simulink model "nonlinear_dynamics_block"  (R2024b)
settings: Solver=VariableStepAuto  StartTime=0.0  StopTime=10.0  RelTol=1e-3
undefined symbols (not defined in the file): K
settings Model: Creator=kaleb  LastModifiedBy=kaleb
settings DataIOCC: ExternalInput=getinputstruct(op_trim1)  InitialState=getstatestruct(op_trim1)

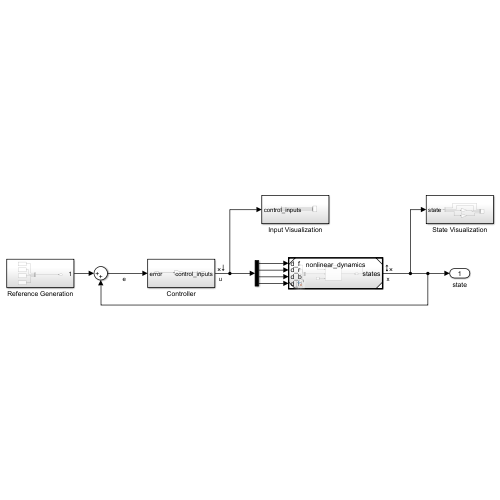
[thumbnail: Simulink's stored preview of the top-level diagram]
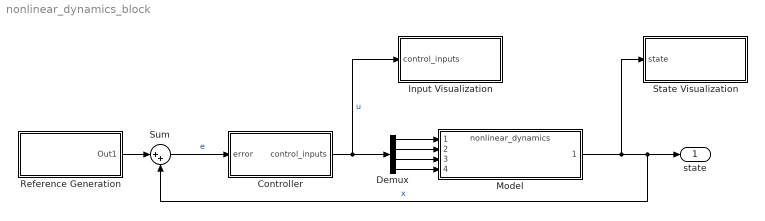
== system nonlinear_dynamics_block ==
  Controller : Subsystem
  Demux : Demux
  Input Visualization : Subsystem
  Model : ModelReference  ModelNameDialog=nonlinear_dynamics.slx  ModelReferenceVersion=1.2
  Reference Generation : Subsystem
  State Visualization : Subsystem
  Sum : Sum  Inputs=|++
  state : Outport
  wires:
  Sum/1 -> Controller/1(error)  "e"
  Reference Generation/1(Out1) -> Sum/1
  Model/1 -> State Visualization/1(state), state/1, Sum/2  "x"
  Controller/1(control_inputs) -> Input Visualization/1(control_inputs), Demux/1  "u"
  Demux/3 -> Model/3
  Demux/4 -> Model/4
  Demux/2 -> Model/2
  Demux/1 -> Model/1

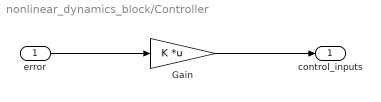
== system nonlinear_dynamics_block/Controller ==
  error : Inport
  Gain : Gain  Gain=K  Multiplication=Matrix(K*u)
  control_inputs : Outport
  wires:
  error/1 -> Gain/1
  Gain/1 -> control_inputs/1

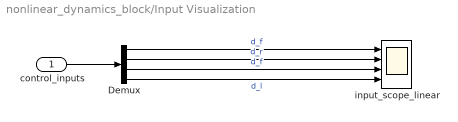
== system nonlinear_dynamics_block/Input Visualization ==
  control_inputs : Inport
  Demux : Demux
  input_scope_linear : Scope  NumInputPorts=4
  wires:
  Demux/4 -> input_scope_linear/4  "d_l"
  Demux/1 -> input_scope_linear/1  "d_f"
  Demux/2 -> input_scope_linear/2  "d_r"
  Demux/3 -> input_scope_linear/3  "d_f"
  control_inputs/1 -> Demux/1

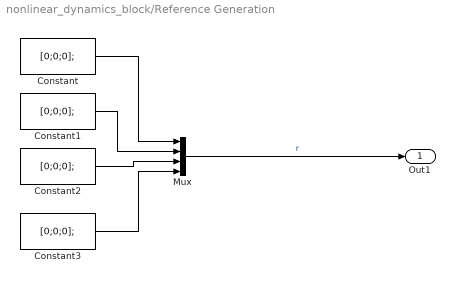
== system nonlinear_dynamics_block/Reference Generation ==
  Constant{,1..3} (4 alike) : Constant  Value=[0;0;0];
  Mux : Mux
  Out1 : Outport
  wires:
  Mux/1 -> Out1/1  "r"
  Constant/1 -> Mux/1
  Constant1/1 -> Mux/2
  Constant2/1 -> Mux/3
  Constant3/1 -> Mux/4

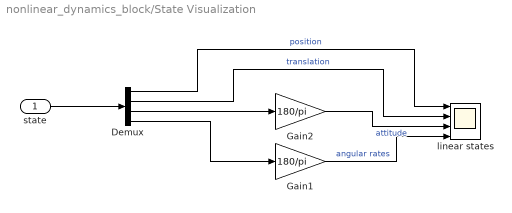
== system nonlinear_dynamics_block/State Visualization ==
  state : Inport
  Demux : Demux
  Gain1 : Gain  Gain=180/pi
  Gain2 : Gain  Gain=180/pi
  linear states : Scope  NumInputPorts=4
  wires:
  state/1 -> Demux/1
  Demux/4 -> Gain1/1
  Demux/1 -> linear states/1  "position"
  Gain2/1 -> linear states/3  "attitude"
  Demux/3 -> Gain2/1
  Gain1/1 -> linear states/4  "angular rates"
  Demux/2 -> linear states/2  "translation"
